simulink model "etrs_sf"  (R2023b)
settings: Solver=VariableStepAuto  StartTime=0.0  StopTime=10.0  RelTol=1e-3
settings Model: Creator=EndUser  LastModifiedBy=EndUser

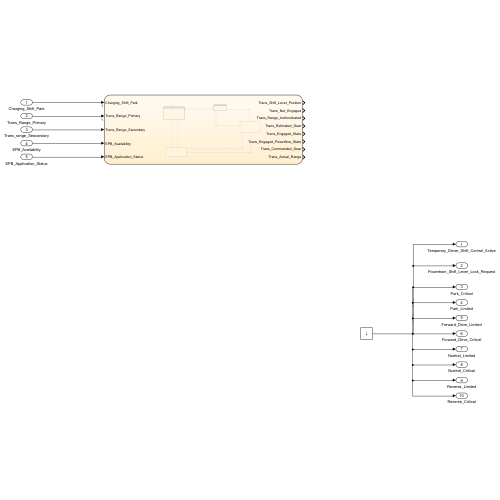
[thumbnail: Simulink's stored preview of the top-level diagram]
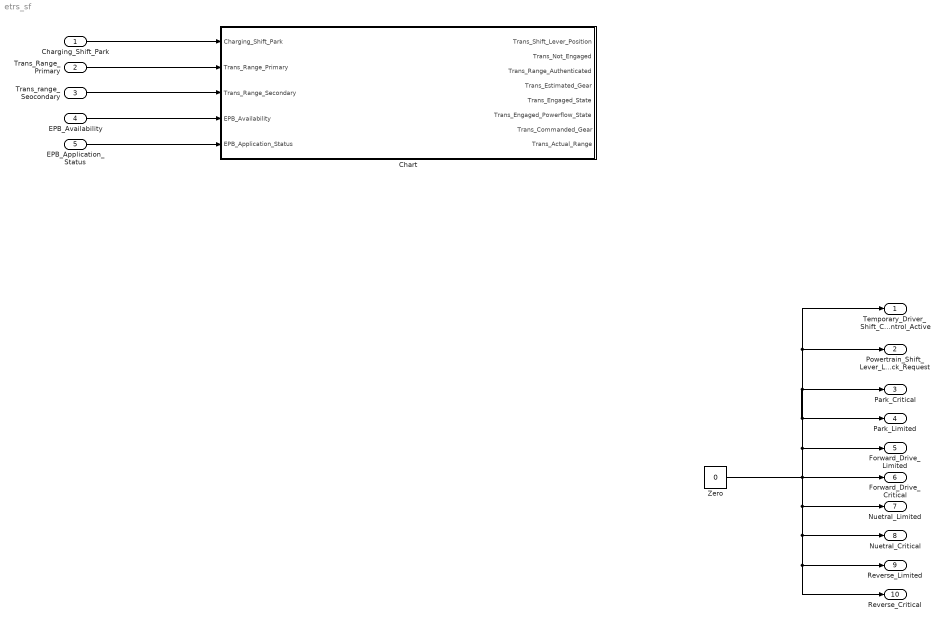
== system etrs_sf ==
  Charging_Shift_Park : Inport
  Trans_Range_Primary : Inport  Port=2
  Trans_range_Seocondary : Inport  Port=3
  EPB_Availability : Inport  Port=4
  EPB_Application_Status : Inport  Port=5
  Chart : Stateflow chart  TreatAsAtomicUnit=on
  Zero : Constant  Value=0  OutDataTypeStr=Inherit: Inherit via back propagation
  Temporary_Driver_Shift_Control_Active : Outport
  Powertrain_Shift_Lever_Lock_Request : Outport  Port=2
  Park_Critical : Outport  Port=3
  Park_Limited : Outport  Port=4
  Forward_Drive_Limited : Outport  Port=5
  Forward_Drive_Critical : Outport  Port=6
  Nuetral_Limited : Outport  Port=7
  Nuetral_Critical : Outport  Port=8
  Reverse_Limited : Outport  Port=9
  Reverse_Critical : Outport  Port=10
  wires:
  Zero/1 -> Temporary_Driver_Shift_Control_Active/1, Powertrain_Shift_Lever_Lock_Request/1, Park_Critical/1, Nuetral_Limited/1, Reverse_Limited/1, Reverse_Critical/1, Nuetral_Critical/1, Forward_Drive_Critical/1, Forward_Drive_Limited/1, Park_Limited/1
  Trans_range_Seocondary/1 -> Chart/3(Trans_Range_Secondary)
  Charging_Shift_Park/1 -> Chart/1(Charging_Shift_Park)
  Trans_Range_Primary/1 -> Chart/2(Trans_Range_Primary)
  EPB_Availability/1 -> Chart/4(EPB_Availability)
  EPB_Application_Status/1 -> Chart/5(EPB_Application_Status)

== stateflow chart etrs_sf/Chart ==
  state Nuetral
    entry:
    Trans_Actual_Range == Nuetral_Position;
    Trans_Range_Authenticated == Nuetral;
    Trans_Shift_Lever_Position == Nuetral_Range;
    Trans_Estimated_Gear == Nuetral_Gear;
    Trans_Commanded_Gear == Nuetral_Gear;
    Trans_Engaged_State == Trans_Not_Engaged;
    Trans_Engaged_Powerflow_State == No_Powerflow;
  state Park
    entry:
    Trans_Range_Authenticated == Park;
    Trans_Shift_Lever_Position == Park_Range;
    Trans_Estimated_Gear == Park_Gear;
    Trans_Commanded_Gear == Park_Gear;
    Trans_Engaged_State == Trans_Not_Engaged;
    Trans_Engaged_Powerflow_State == No_Powerflow;
    (default) -> (junction 68) : % Actual_Range
    (junction 68) -> (junction 69) [order 1] : [EPB_Application_Status == Engaged]
    (junction 68) -> (junction 70) [order 2] : {Trans_Actual_Range == Nuetral_Position}
    (junction 69) -> (junction 71) : {Trans_Actual_Range == Park_Position}
    (junction 71) -> (junction 70)
    (junction 70) -> (junction 72)
  state Drive
    entry:
    Trans_Actual_Range == First_Drive_Position;
    Trans_Range_Authenticated == Drive;
    Trans_Shift_Lever_Position == Forward_Range;
    Trans_Estimated_Gear == CVT_Forward_Gear;
    Trans_Commanded_Gear == CVT_Forward_Gear;
    Trans_Engaged_State == Trans_Engaged_Forward;
    Trans_Engaged_Powerflow_State == Forward_Engaged;
  state Reverse
    entry:
    Trans_Actual_Range == Reverse_Position;
    Trans_Range_Authenticated == Reverse;
    Trans_Shift_Lever_Position == Reverse_Range;
    Trans_Estimated_Gear == Reverse_Gear;
    Trans_Commanded_Gear == Reverse_Gear;
    Trans_Engaged_State == Trans_Engaged_Reverse;
    Trans_Engaged_Powerflow_State == Reverse_Engaged;
  (default) -> Park
  Park -> Nuetral [order 1] : [(Trans_Range_Primary== Nuetral || Trans_Range_Primary== Drive) && Charging_Shift_Park == 0]
  Nuetral -> (junction 80) [order 1] : [Trans_Range_Primary== Drive]
  Nuetral -> Park [order 2] : [(Trans_Range_Primary== Park || Charging_Shift_Park == 1) && EPB_Availability == Available ]
  (junction 80) -> Drive
  (junction 84) -> Nuetral
  Reverse -> Park [order 2] : [(Trans_Range_Primary== Park || Charging_Shift_Park == 1) && EPB_Availability == Available]
  Park -> Reverse [order 2] : [Trans_Range_Primary== Reverse && Charging_Shift_Park == 0 ]
  Drive -> (junction 84) [order 2] : [Trans_Range_Primary== Nuetral || ((Trans_Range_Primary== Park || Charging_Shift_Park == 1) && EPB_Availability == Available )]
  Drive -> (junction 87) [order 1] : [Trans_Range_Primary== Reverse]
  (junction 86) -> Drive
  (junction 87) -> Reverse
  Reverse -> (junction 86) [order 1] : [Trans_Range_Primary== Drive]
  data: Charging_Shift_Park input; Trans_Range_Primary input; Reverse local; Park_Range local; Park_Position local; Park_Gear local; Park local; Nuetral_Range local; Nuetral_Position local; Nuetral_Gear local; Nuetral local; No_Powerflow local; Drive local; Trans_Shift_Lever_Position output; Trans_Not_Engaged output; Trans_Range_Authenticated output; Trans_Estimated_Gear output; Trans_Engaged_State output; Trans_Engaged_Powerflow_State output; Trans_Commanded_Gear output; Trans_Engaged_Reverse local; Trans_Engaged_Forward local; Reverse_Range local; Reverse_Gear local; Reverse_Engaged local; Forward_Range local; Forward_Engaged local; CVT_Forward_Gear local; Trans_Range_Secondary input; Trans_Actual_Range output; Reverse_Position local; First_Drive_Position local; Engaged local; EPB_Availability input; EPB_Application_Status input; Available local
